simulink library "DynamicsInput_Lib"  (R2019b)
settings: Solver=VariableStepAuto  StartTime=0.0  StopTime=10.0  RelTol=1e-3
undefined symbols (not defined in the file): BrakingForce, FreezeDynamics, LockedAxle, SandingApplied, TractionForce, WheelFlat
settings Model: Creator=rleighton  LastModifiedBy=mondt
settings DebuggingCC: ArithmeticOperatorsInVariantConditions=warning
settings SFSimCC: SimUseLocalCustomCode=off  CustomCodeUndefinedFunction=UseInterfaceOnly
settings RTWCC: RTWUseLocalCustomCode=off

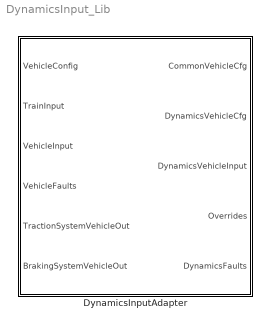
== system DynamicsInput_Lib ==
  DynamicsInputAdapter : Subsystem  TreatAsAtomicUnit=on  SystemSampleTime=0.01

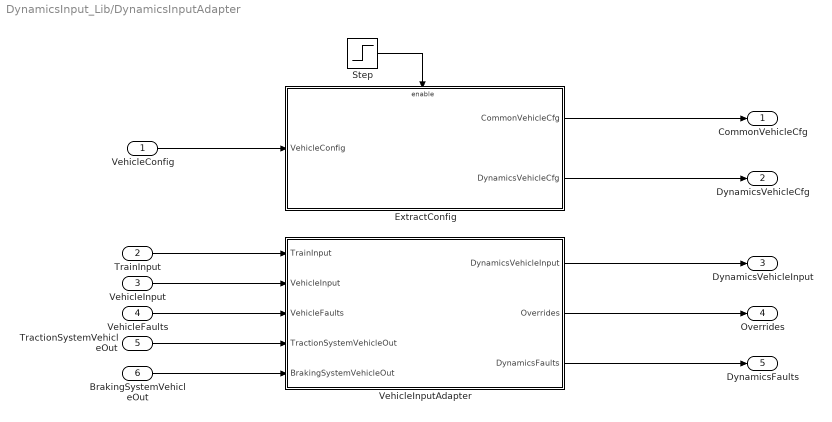
== system DynamicsInput_Lib/DynamicsInputAdapter ==
  VehicleConfig : Inport
  TrainInput : Inport  Port=2
  VehicleInput : Inport  Port=3
  VehicleFaults : Inport  Port=4
  TractionSystemVehicleOut : Inport  Port=5
  BrakingSystemVehicleOut : Inport  Port=6
  ExtractConfig : Subsystem
  Step : Step  Before=1  After=0
  VehicleInputAdapter : Subsystem
  CommonVehicleCfg : Outport  VectorParamsAs1DForOutWhenUnconnected=off
  DynamicsVehicleCfg : Outport  Port=2  VectorParamsAs1DForOutWhenUnconnected=off
  DynamicsVehicleInput : Outport  Port=3  VectorParamsAs1DForOutWhenUnconnected=off
  Overrides : Outport  Port=4  VectorParamsAs1DForOutWhenUnconnected=off
  DynamicsFaults : Outport  Port=5  VectorParamsAs1DForOutWhenUnconnected=off
  wires:
  VehicleInputAdapter/3(DynamicsFaults) -> DynamicsFaults/1
  VehicleInputAdapter/2(Overrides) -> Overrides/1
  VehicleInputAdapter/1(DynamicsVehicleInput) -> DynamicsVehicleInput/1
  VehicleFaults/1 -> VehicleInputAdapter/3(VehicleFaults)
  Step/1 -> ExtractConfig/Enable
  ExtractConfig/2(DynamicsVehicleCfg) -> DynamicsVehicleCfg/1
  ExtractConfig/1(CommonVehicleCfg) -> CommonVehicleCfg/1
  VehicleConfig/1 -> ExtractConfig/1(VehicleConfig)
  BrakingSystemVehicleOut/1 -> VehicleInputAdapter/5(BrakingSystemVehicleOut)
  TractionSystemVehicleOut/1 -> VehicleInputAdapter/4(TractionSystemVehicleOut)
  VehicleInput/1 -> VehicleInputAdapter/2(VehicleInput)
  TrainInput/1 -> VehicleInputAdapter/1(TrainInput)

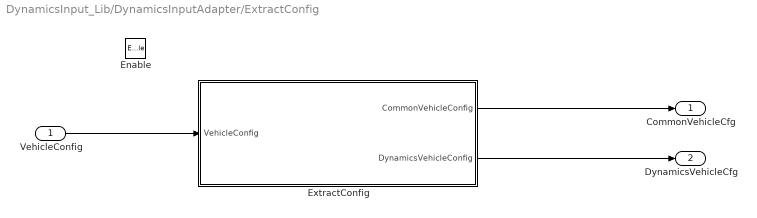
== system DynamicsInput_Lib/DynamicsInputAdapter/ExtractConfig ==
  VehicleConfig : Inport
  Enable : EnablePort
  ExtractConfig : Subsystem
  CommonVehicleCfg : Outport  VectorParamsAs1DForOutWhenUnconnected=off
  DynamicsVehicleCfg : Outport  Port=2  VectorParamsAs1DForOutWhenUnconnected=off
  wires:
  VehicleConfig/1 -> ExtractConfig/1(VehicleConfig)
  ExtractConfig/1(CommonVehicleConfig) -> CommonVehicleCfg/1
  ExtractConfig/2(DynamicsVehicleConfig) -> DynamicsVehicleCfg/1

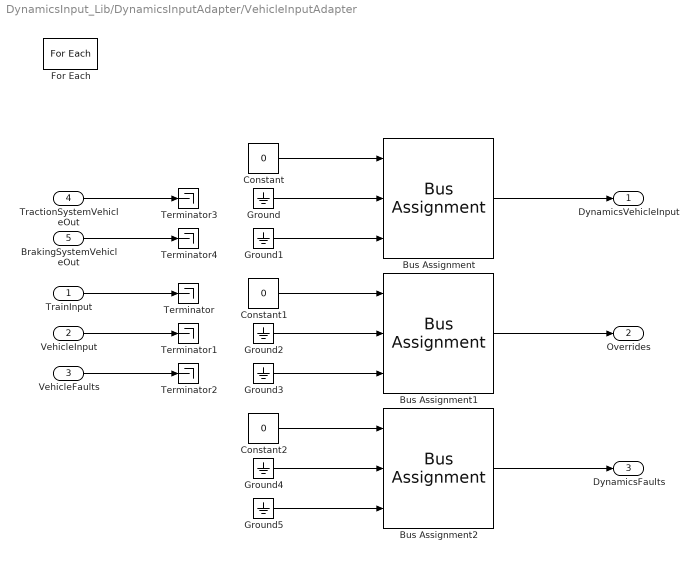
== system DynamicsInput_Lib/DynamicsInputAdapter/VehicleInputAdapter ==
  TrainInput : Inport
  VehicleInput : Inport  Port=2  Partition=on  PartitionDimension=1  PartitionWidth=1  PartitionOffset=0
  VehicleFaults : Inport  Port=3  Partition=on  PartitionDimension=1  PartitionWidth=1  PartitionOffset=0
  TractionSystemVehicleOut : Inport  Port=4  Partition=on  PartitionDimension=1  PartitionWidth=1  PartitionOffset=0
  BrakingSystemVehicleOut : Inport  Port=5  Partition=on  PartitionDimension=1  PartitionWidth=1  PartitionOffset=0
  Bus Assignment : BusAssignment  AssignedSignals=TractionForce,BrakingForce
  Bus Assignment1 : BusAssignment  AssignedSignals=FreezeDynamics,SandingApplied
  Bus Assignment2 : BusAssignment  AssignedSignals=LockedAxle,WheelFlat
  Constant : Constant  Value=0  OutDataTypeStr=Bus: BD_TrainDynamics_In_Vehicle
  Constant1 : Constant  Value=0  OutDataTypeStr=Bus: BD_TrainDynamics_In_Vehicle_Overrides
  Constant2 : Constant  Value=0  OutDataTypeStr=Bus: BD_TrainDynamics_In_Vehicle_Faults
  For Each : ForEach  DisableCoverage=on
  Ground{,1..5} (6 alike) : Ground
  Terminator{,1..4} (5 alike) : Terminator
  DynamicsVehicleInput : Outport  ConcatenationDimension=1  VectorParamsAs1DForOutWhenUnconnected=off
  Overrides : Outport  Port=2  ConcatenationDimension=1  VectorParamsAs1DForOutWhenUnconnected=off
  DynamicsFaults : Outport  Port=3  ConcatenationDimension=1  VectorParamsAs1DForOutWhenUnconnected=off
  wires:
  Bus Assignment2/1 -> DynamicsFaults/1
  Constant2/1 -> Bus Assignment2/1
  Ground5/1 -> Bus Assignment2/3
  Ground4/1 -> Bus Assignment2/2
  Bus Assignment1/1 -> Overrides/1
  Ground2/1 -> Bus Assignment1/2
  Ground3/1 -> Bus Assignment1/3
  Constant1/1 -> Bus Assignment1/1
  Ground1/1 -> Bus Assignment/3
  Ground/1 -> Bus Assignment/2
  Bus Assignment/1 -> DynamicsVehicleInput/1
  Constant/1 -> Bus Assignment/1
  BrakingSystemVehicleOut/1 -> Terminator4/1
  TractionSystemVehicleOut/1 -> Terminator3/1
  VehicleFaults/1 -> Terminator2/1
  VehicleInput/1 -> Terminator1/1
  TrainInput/1 -> Terminator/1

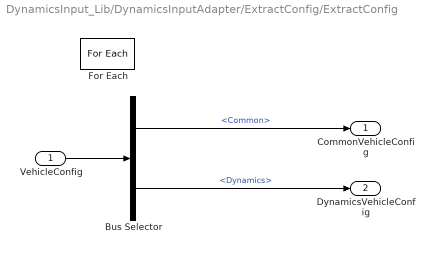
== system DynamicsInput_Lib/DynamicsInputAdapter/ExtractConfig/ExtractConfig ==
  VehicleConfig : Inport  Partition=on  PartitionDimension=1  PartitionWidth=1  PartitionOffset=0  BusOutputAsStruct=on
  Bus Selector : BusSelector  OutputSignals=Common,Dynamics
  For Each : ForEach  DisableCoverage=on
  CommonVehicleConfig : Outport  ConcatenationDimension=1  VectorParamsAs1DForOutWhenUnconnected=off
  DynamicsVehicleConfig : Outport  Port=2  ConcatenationDimension=1  VectorParamsAs1DForOutWhenUnconnected=off
  wires:
  Bus Selector/2 -> DynamicsVehicleConfig/1  "<Dynamics>"
  Bus Selector/1 -> CommonVehicleConfig/1  "<Common>"
  VehicleConfig/1 -> Bus Selector/1
